simulink model "Vehicle"  (R2018a)
settings: Solver=VariableStepAuto  StartTime=0.0  StopTime=10.0  RelTol=1e-3
values from neighbouring files (symbols this model uses):
  Cf = 1.3    [data_vehicle.m]    (also in forwardPropagate.m = 19000; matlab.mat; myVehicle.m = this.CF; testMotionPlanner.mat)
  Cr = 1.3    [data_vehicle.m]    (also in forwardPropagate.m = 33000; matlab.mat; myVehicle.m = this.CR; testMotionPlanner.mat)
  Iz = 2875    [forwardPropagate.m]    (also in matlab.mat; myVehicle.m = this.IZ)
  lf = 1    [data_vehicle.m]    (also in forwardPropagate.m = 1.2; matlab.mat; myVehicle.m = this.LF; testMotionPlanner.mat)
  lr = l-lf    (= 1.7)    [data_vehicle.m]    (also in forwardPropagate.m = 1.6; matlab.mat; myVehicle.m = this.LR; testMotionPlanner.mat)
  m = 1600    [data_vehicle.m]    (also in forwardPropagate.m = 1575; matlab.mat; myVehicle.m = this.M; testMotionPlanner.mat)
  x0_ego = from(1)    [forwardPropagate.m]    (also in matlab.mat = 1.6; testMotionPlanner.mat = 1.6)
  xdot0 = from(4)    [forwardPropagate.m]
  y0_ego = from(2)    [forwardPropagate.m]    (also in matlab.mat = -1.8; testMotionPlanner.mat = -1.8)
  yaw0_ego = from(3)    [forwardPropagate.m]    (also in matlab.mat = -4.07806561609; testMotionPlanner.mat = -4.07806561609)
  yawrate0 = from(6)    [forwardPropagate.m]
libraries: autolibshared x1
settings Model: Creator=jdrjk  LastModifiedBy=jdrjk
settings DataIOCC: SaveCompleteFinalSimState=on  SignalLogging=off  DSMLogging=off

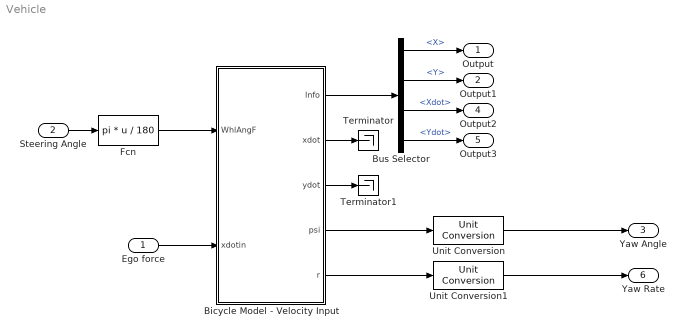
== system Vehicle ==
  Ego force : Inport
  Steering Angle : Inport  Port=2
  Bicycle Model - Velocity Input : Subsystem  AncestorBlock=autolibshared/Bicycle Model - Velocity Input  mask(Vehicle Body 3DOF Lateral){trackMode=Single (bicycle), inputMode=External longitudinal forces, frontSteerMode=on, rearSteerMode=off, windMode=off, muMode=off, extFMode=off, extMMode=off, aMode=3, NF=2, NR=2, m=m, a=lf, b=lr, h=0.35, X_o=x0_ego, xdot_o=xdot0, CalphaMode=off, sigmaMode=on, w=[1.4,1.4], Cy_f=Cf, Cy_r=Cr, sigma_f=.1, sigma_r=.1, alpha_f_brk=[-.1 .1], Cy_f_data=[-9e3 9e3], alpha_r_brk=[-.1 .1], Cy_r_data=[-9e3 9e3], Y_o=y0_ego, ydot_o=0, Izz=Iz, psi_o=yaw0_ego*pi/180, r_o=yawrate0*pi/180, Af=2, Cd=.3, Cl=.1, Cpm=.1, beta_w=[0:0.01:0.3], Cs=[0:0.03:0.9], Cym=[0:0.01:0.3], Pabs=101325, Tair=273, g=9.81, mu=1, xdot_tol=.01, Fznom=5000, Fxtire_sat=1e6, Fytire_sat=1e6}
      mask prompts: trackMode "Vehicle track:"; inputMode "Axle forces:"; frontSteerMode "Front wheel steering"; rearSteerMode "Rear wheel steering"; windMode "External wind"; muMode "External friction"; extFMode "External forces"; extMMode "External moments"; NF "Number of wheels on front axle, NF [-]:"; NR "Number of wheels on rear axle, NR [-]:"; m "Vehicle mass, m [kg]:"; a "Longitudinal distance from center of mass to front axle, a [m]:"; b "Longitudinal distance from center of mass to rear axle, b [m]:"; h "Vertical distance from center of mass to axle plane, h [m]:"; X_o "Initial inertial frame longitudinal position, X_o [m]:"; xdot_o "Initial longitudinal velocity, xdot_o [m/s]:"; CalphaMode "Mapped corner stiffness:"; sigmaMode "Include relaxation length dynamics:"; w "Track width, w [m]:"; Cy_f "Front tire corner stiffness, Cy_f [N/rad]:"; Cy_r "Rear tire axle corner stiffness, Cy_r [N/rad]:"; sigma_f "Front tire(s) relaxation length, sigma_f [m]:"; sigma_r "Rear tire(s) relaxation length, sigma_r [m]:"; alpha_f_brk "Front axle slip angle breakpoints, alpha_f_brk [rad]:"; Cy_f_data "Front axle corner data, Cy_f_data [N/rad]:"; alpha_r_brk "Rear axle slip angle breakpoints, alpha_r_brk [rad]:"; Cy_r_data "Rear axle corner data, Cy_r_data [N/rad]:"; Y_o "Initial inertial frame lateral displacement, Y_o [m]:"; ydot_o "Initial lateral velocity, ydot_o [m/s]:"; Izz "Yaw polar inertia, Izz [kg*m^2]:"; psi_o "Initial yaw angle, psi_o [rad]:"; r_o "Initial yaw rate, r_o [rad/s]:"; Af "Longitudinal drag area, Af [m^2]:"; Cd "Longitudinal drag coefficient, Cd [-]:"; Cl "Longitudinal lift coefficient, Cl [-]:"; Cpm "Longitudinal drag pitch moment, Cpm [-]:"; beta_w "Relative wind angle vector, beta_w [rad]:"; Cs "Side force coefficient vector, Cs [-]:"; Cym "Yaw moment coefficient vector, Cym [-]:"; Pabs "Absolute pressure, Pabs [Pa]:"; Tair "Air temperature, Tair [K]:"; g "Gravitational acceleration, g [m/s^2]:"; mu "Nominal friction scaling factor, mu [-]:"; xdot_tol "Longitudinal velocity tolerance, xdot_tol [m/s]:"; Fznom "Nominal normal force, Fznom [N]:"; Fxtire_sat "Longitudinal force limit, Fxtire_sat [N]:"; Fytire_sat "Lateral force limit, Fytire_sat [N]:"
      mask help: Implements a 3 DOF rigid two-axle vehicle body model to calculate longitudinal, lateral, and yaw motion. Accounts for body mass, aerodynamic drag, and weight distribution between the axles due to acceleration and steering.
      mask init:
      | [~]=autosharedicon('autolibvehdyn3doflatr',gcb,0);
      mask Help: eval('autosharedhelp(''vbbicycle'')');
      mask TypeOptions trackMode: Single (bicycle) | Dual
      mask Callback trackMode: %[~]=vehdynicon('vehdynliblat3dof',gcb,5);
      mask TypeOptions inputMode: External longitudinal velocity | External longitudinal forces | External forces
      mask Callback inputMode: %[~]=vehdynicon('vehdynliblat3dof',gcb,1);
      mask Callback muMode: %[~]=vehdynicon('vehdynliblat3dof',gcb,2);
      mask Callback CalphaMode: %[~]=vehdynicon('vehdynliblat3dof',gcb,3);
      mask Callback sigmaMode: %[~]=vehdynicon('vehdynliblat3dof',gcb,4);
      mask DialogControl blockConfig Prompt: Block Options:
      mask DialogControl ParameterGroupVar Prompt: Vehicle Parameters
      mask DialogControl LongPanel Prompt: Longitudinal
      mask DialogControl LatPanel Prompt: Lateral
      mask DialogControl YawPanel Prompt: Yaw
      mask DialogControl AeroParams Prompt: Aerodynamic
      mask DialogControl EnviroPanel Prompt: Environment
      mask DialogControl SimPanel Prompt: Simulation
      mask Display:
      | try
      |     IconInfo = autosharedicon('autolibvehdyn3doflatr',gcb,8);
      | 
      |     image(IconInfo.image, IconInfo.position);
      | 
      |     for i = 1:numel(IconInfo.lconn)
      |         port_label('lconn', i, IconInfo.lconn{i})
      |     end
      | 
      |     for j = 1:numel(IconInfo.rconn)
      |         port_label('rconn', j, IconInfo.rconn{j})
      |     end
      | 
      |     for k = 1:numel(IconInfo.input)
      |         port_label('input', k, IconInfo.input{k})
      |     end
      | 
      |     for m = 1:numel(IconInfo.output)
      |         port_label('output', m, IconInfo.output{m})
      |     end
      | catch
      |     fprintf('Vehicle Body \n 3DOF Lateral')
      | end
  Bus Selector : BusSelector  OutputSignals=InertFrm.FrntAxl.Disp.X,InertFrm.FrntAxl.Disp.Y,InertFrm.FrntAxl.Vel.Xdot,InertFrm.FrntAxl.Vel.Ydot
  Fcn : Fcn  Expr=pi * u / 180
  Terminator : Terminator
  Terminator1 : Terminator
  Unit Conversion : UnitConversion  OutputType=Inherit: Inherit via back propagation
  Unit Conversion1 : UnitConversion  OutputType=Inherit: Inherit via back propagation
  Output : Outport
  Output1 : Outport  Port=2
  Yaw Angle : Outport  Port=3  Unit=deg
  Output2 : Outport  Port=4
  Output3 : Outport  Port=5
  Yaw Rate : Outport  Port=6  Unit=degree/s
  wires:
  Bus Selector/4 -> Output3/1  "<Ydot>"
  Ego force/1 -> Bicycle Model - Velocity Input/2(xdotin)
  Bicycle Model - Velocity Input/3(ydot) -> Terminator1/1
  Bicycle Model - Velocity Input/2(xdot) -> Terminator/1
  Bus Selector/1 -> Output/1  "<X>"
  Bus Selector/3 -> Output2/1  "<Xdot>"
  Unit Conversion/1 -> Yaw Angle/1
  Bicycle Model - Velocity Input/5(r) -> Unit Conversion1/1
  Bicycle Model - Velocity Input/1(Info) -> Bus Selector/1
  Unit Conversion1/1 -> Yaw Rate/1
  Fcn/1 -> Bicycle Model - Velocity Input/1(WhlAngF)
  Bicycle Model - Velocity Input/4(psi) -> Unit Conversion/1
  Bus Selector/2 -> Output1/1  "<Y>"
  Steering Angle/1 -> Fcn/1

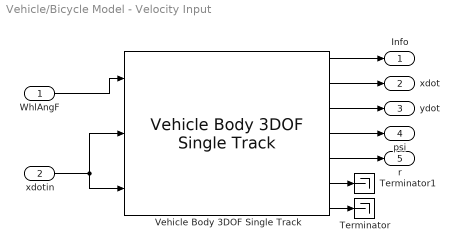
== system Vehicle/Bicycle Model - Velocity Input ==
  WhlAngF : Inport  Unit=rad
  xdotin : Inport  Port=2  Unit=N
  Terminator : Terminator
  Terminator1 : Terminator
  Vehicle Body 3DOF Single Track : autolibshared/Vehicle Body 3DOF Single Track  trackMode=Single (bicycle)  inputMode=External longitudinal forces  frontSteerMode=on  rearSteerMode=off  windMode=off  muMode=off  extFMode=off  extMMode=off  aMode=3  NF=NF  NR=NR  m=m  a=a  b=b  h=h  X_o=X_o  xdot_o=xdot_o  CalphaMode=off  sigmaMode=on  w=[1.4,1.4]  Cy_f=Cy_f  Cy_r=Cy_r  sigma_f=.1  sigma_r=.1  alpha_f_brk=[-.1 .1]  Cy_f_data=[-9e3 9e3]  alpha_r_brk=[-.1 .1]  Cy_r_data=[-9e3 9e3]  Y_o=Y_o  ydot_o=ydot_o  Izz=Izz  psi_o=psi_o  r_o=r_o  Af=Af  Cd=Cd  Cl=Cl  Cpm=Cpm  beta_w=beta_w  Cs=Cs  Cym=Cym  Pabs=Pabs  Tair=Tair  g=g  mu=mu  xdot_tol=xdot_tol  Fznom=Fznom  Fxtire_sat=Fxtire_sat  Fytire_sat=Fytire_sat
      settings: SourceProductName=Powertrain Blockset  SourceProductBaseCode=PW
  Info : Outport
  xdot : Outport  Port=2
  ydot : Outport  Port=3
  psi : Outport  Port=4
  r : Outport  Port=5
  wires:
  Vehicle Body 3DOF Single Track/1 -> Info/1
  Vehicle Body 3DOF Single Track/4 -> psi/1
  WhlAngF/1 -> Vehicle Body 3DOF Single Track/1
  Vehicle Body 3DOF Single Track/2 -> xdot/1
  Vehicle Body 3DOF Single Track/3 -> ydot/1
  Vehicle Body 3DOF Single Track/5 -> r/1
  Vehicle Body 3DOF Single Track/6 -> Terminator1/1
  xdotin/1 -> Vehicle Body 3DOF Single Track/3, Vehicle Body 3DOF Single Track/2
  Vehicle Body 3DOF Single Track/7 -> Terminator/1
